simulink model "testing_time_net_3layers"  (R2018b)
settings: Solver=VariableStepAuto  StartTime=0.0  StopTime=10.0  RelTol=1e-3
libraries: neural x97
(part 2 of 6)

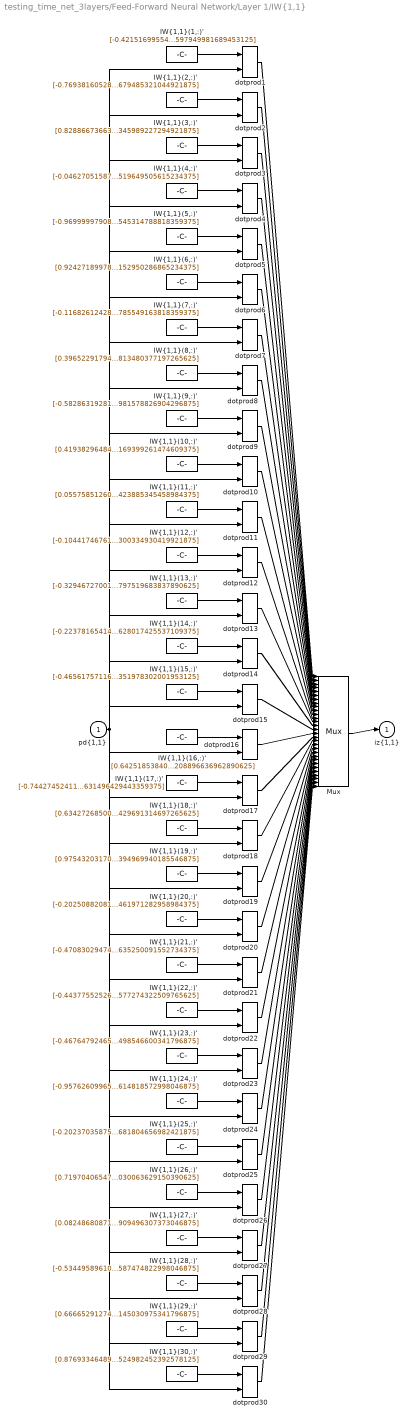
== system testing_time_net_3layers/Feed-Forward Neural Network/Layer 1/IW{1,1} ==
  "pd{1,1}" : Inport  PortDimensions=10
      mask Display: e = 0.06;c1 = [120 230 180]/255;c2 = ([120 230 180]+0)/(256+128);c3 = ([120 230 180]+128)/(256+128);patch([0 1 1 0],[0 0 1 1],c1);patch([0 1 1 1-e 1-e 0+e],[0 0 1 1-e 0+e 0+e],c2);patch([0 0 1 1-e 0+e 0+e],[0 1 1 1-e 1-e 0+e],c3);plot([0 1 1 0 0],[0 0 1 1 0]);
  "IW{1,1}(1,:)'" : Constant  Value=[-0.421516995547151440693056656527915038168430328369140625;-0.78331730650782827041211930918507277965545654296875;0.87573894753330805418300997189362533390522003173828125;0.12417975566875194548543959172093309462070465087890625;-0.1892164229878487702318778929111431352794170379638671875;0.77197968809492589770115955616347491741180419921875;-0.162179356745227154501520772100775502622127532958984375;-0.47501513253533367286962629805202595889568328857421875;0.361899777531295041566039571989676915109157562255859375;-1.0678850199978360269170707397279329597949981689453125]
      mask Display: e = 0.06;c1 = [120 150 230]/255;c2 = ([120 150 230]+0)/383;c3 = ([120 150 230]+128)/383;patch([0 1 1 0],[0 0 1 1],c1);patch([0 1 1 1-e 1-e 0+e],[0 0 1 1-e 0+e 0+e],c2);patch([0 0 1 1-e 0+e 0+e],[0 1 1 1-e 1-e 0+e],c3);plot([0 1 1 0 0],[0 0 1 1 0]);disp('Weights');
  "IW{1,1}(10,:)'" : Constant  Value=[0.419382964847384187567769231463898904621601104736328125;-1.10662440705737896706750689190812408924102783203125;-0.520362222704379373539040898322127759456634521484375;-0.7192359088296094160597249356214888393878936767578125;-1.00725625065982793415741980425082147121429443359375;0.21548425562980089154052620870061218738555908203125;0.381727115430177843524717218315345235168933868408203125;0.04936193217574691427529387510730884969234466552734375;-0.430557268169915463573715896927751600742340087890625;0.22991864804537021083064018966979347169399261474609375]
      mask Display: e = 0.06;c1 = [120 150 230]/255;c2 = ([120 150 230]+0)/383;c3 = ([120 150 230]+128)/383;patch([0 1 1 0],[0 0 1 1],c1);patch([0 1 1 1-e 1-e 0+e],[0 0 1 1-e 0+e 0+e],c2);patch([0 0 1 1-e 0+e 0+e],[0 1 1 1-e 1-e 0+e],c3);plot([0 1 1 0 0],[0 0 1 1 0]);disp('Weights');
  "IW{1,1}(11,:)'" : Constant  Value=[0.055758512605714904974973933349247090518474578857421875;-0.81841828037387120975409970924374647438526153564453125;1.1440676666439248965190245144185610115528106689453125;-0.36136848687608680297245200563338585197925567626953125;-0.86626831394689973731004783985554240643978118896484375;0.0149492584043128019788415627999711432494223117828369140625;-0.048457932577146568819959071561243035830557346343994140625;0.1490262934767860036888720287606702186167240142822265625;-0.2238428092966452676026989365709596313536167144775390625;0.80848234625489057147973426253884099423885345458984375]
      mask Display: e = 0.06;c1 = [120 150 230]/255;c2 = ([120 150 230]+0)/383;c3 = ([120 150 230]+128)/383;patch([0 1 1 0],[0 0 1 1],c1);patch([0 1 1 1-e 1-e 0+e],[0 0 1 1-e 0+e 0+e],c2);patch([0 0 1 1-e 0+e 0+e],[0 1 1 1-e 1-e 0+e],c3);plot([0 1 1 0 0],[0 0 1 1 0]);disp('Weights');
  "IW{1,1}(12,:)'" : Constant  Value=[-0.10441746761245880581459033464852836914360523223876953125;-0.11643946018543309406378938319903681986033916473388671875;0.1902729302910009800964274973011924885213375091552734375;0.469215077641359223914463427718146704137325286865234375;0.06023180084088856911517240178000065498054027557373046875;-1.097601095565966744516117614693939685821533203125;-0.19260021082754497090405720882699824869632720947265625;-0.95631655884358857111493534830515272915363311767578125;0.33607616325035305493429405032657086849212646484375;0.243167221789594101277742765887524001300334930419921875]
      mask Display: e = 0.06;c1 = [120 150 230]/255;c2 = ([120 150 230]+0)/383;c3 = ([120 150 230]+128)/383;patch([0 1 1 0],[0 0 1 1],c1);patch([0 1 1 1-e 1-e 0+e],[0 0 1 1-e 0+e 0+e],c2);patch([0 0 1 1-e 0+e 0+e],[0 1 1 1-e 1-e 0+e],c3);plot([0 1 1 0 0],[0 0 1 1 0]);disp('Weights');
  "IW{1,1}(13,:)'" : Constant  Value=[-0.32946727001318809602281589832273311913013458251953125;-0.59573828714480148160959060987806878983974456787109375;0.047375503865274802561824429858461371622979640960693359375;-0.8972999906601477615453177349991165101528167724609375;0.1344036346182840013785408928015385754406452178955078125;-0.307730158359239336363089023507200181484222412109375;-0.50048527970131839737177870119921863079071044921875;0.5770479702135820065933557998505420982837677001953125;1.0835405192943083907408663435489870607852935791015625;0.00146764010904052756567583770674900733865797519683837890625]
      mask Display: e = 0.06;c1 = [120 150 230]/255;c2 = ([120 150 230]+0)/383;c3 = ([120 150 230]+128)/383;patch([0 1 1 0],[0 0 1 1],c1);patch([0 1 1 1-e 1-e 0+e],[0 0 1 1-e 0+e 0+e],c2);patch([0 0 1 1-e 0+e 0+e],[0 1 1 1-e 1-e 0+e],c3);plot([0 1 1 0 0],[0 0 1 1 0]);disp('Weights');
  "IW{1,1}(14,:)'" : Constant  Value=[-0.2237816541400211300949507631230517290532588958740234375;-0.2255117106004860261236899532377719879150390625;0.66053775807437242750808081837021745741367340087890625;-0.271471723530878839003577240873710252344608306884765625;-0.275504989896624030709659791682497598230838775634765625;1.090081336576464554610765844699926674365997314453125;-1.0836555650409618323237737058661878108978271484375;0.4045819957397511767993592002312652766704559326171875;-0.38831379318925274279905579533078707754611968994140625;0.81705807101285576887761408215737901628017425537109375]
      mask Display: e = 0.06;c1 = [120 150 230]/255;c2 = ([120 150 230]+0)/383;c3 = ([120 150 230]+128)/383;patch([0 1 1 0],[0 0 1 1],c1);patch([0 1 1 1-e 1-e 0+e],[0 0 1 1-e 0+e 0+e],c2);patch([0 0 1 1-e 0+e 0+e],[0 1 1 1-e 1-e 0+e],c3);plot([0 1 1 0 0],[0 0 1 1 0]);disp('Weights');
  "IW{1,1}(15,:)'" : Constant  Value=[-0.465617571164088916990664301920332945883274078369140625;0.20021971547416994585688598817796446382999420166015625;-0.866762424370275397222940227948129177093505859375;-1.15028928445346334541454780264757573604583740234375;0.51764057051554213106925317333661951124668121337890625;0.308597669704476273988547063709120266139507293701171875;-0.37399670770951420895045202996698208153247833251953125;-0.398601119454665531183223947664373554289340972900390625;1.0574802584945477423872262079385109245777130126953125;0.33715076808321076118346582006779499351978302001953125]
      mask Display: e = 0.06;c1 = [120 150 230]/255;c2 = ([120 150 230]+0)/383;c3 = ([120 150 230]+128)/383;patch([0 1 1 0],[0 0 1 1],c1);patch([0 1 1 1-e 1-e 0+e],[0 0 1 1-e 0+e 0+e],c2);patch([0 0 1 1-e 0+e 0+e],[0 1 1 1-e 1-e 0+e],c3);plot([0 1 1 0 0],[0 0 1 1 0]);disp('Weights');
  "IW{1,1}(16,:)'" : Constant  Value=[0.64251853840130268569197369288303889334201812744140625;-0.9103176888822288592706399867893196642398834228515625;0.86486580306804949902499402014655061066150665283203125;-0.802804038444044021360923579777590930461883544921875;-0.0306119017760589258447811999985788133926689624786376953125;0.48642105708010030529209188898676075041294097900390625;-0.32892673265715888231142116637784056365489959716796875;-0.33398839064729857195601425701170228421688079833984375;0.49490021343151535671012197781237773597240447998046875;-0.66415276437832526656990239644073881208896636962890625]
      mask Display: e = 0.06;c1 = [120 150 230]/255;c2 = ([120 150 230]+0)/383;c3 = ([120 150 230]+128)/383;patch([0 1 1 0],[0 0 1 1],c1);patch([0 1 1 1-e 1-e 0+e],[0 0 1 1-e 0+e 0+e],c2);patch([0 0 1 1-e 0+e 0+e],[0 1 1 1-e 1-e 0+e],c3);plot([0 1 1 0 0],[0 0 1 1 0]);disp('Weights');
  "IW{1,1}(17,:)'" : Constant  Value=[-0.7442745241102250997045075564528815448284149169921875;0.8528849176435795431672204358619637787342071533203125;0.1472831429426426919082615540901315398514270782470703125;0.70582238257419860349983764535863883793354034423828125;0.71412598991594522512826870297431014478206634521484375;0.72628375847696113876139634157880209386348724365234375;0.1256024263367492010967652049657772295176982879638671875;-0.46946656479521109428532099627773277461528778076171875;-1.0040813607858349865153968494269065558910369873046875;-0.2292580558718129990491974012911668978631496429443359375]
      mask Display: e = 0.06;c1 = [120 150 230]/255;c2 = ([120 150 230]+0)/383;c3 = ([120 150 230]+128)/383;patch([0 1 1 0],[0 0 1 1],c1);patch([0 1 1 1-e 1-e 0+e],[0 0 1 1-e 0+e 0+e],c2);patch([0 0 1 1-e 0+e 0+e],[0 1 1 1-e 1-e 0+e],c3);plot([0 1 1 0 0],[0 0 1 1 0]);disp('Weights');
  "IW{1,1}(18,:)'" : Constant  Value=[0.63427268500540068263404691606410779058933258056640625;0.59103300526930524494417795722256414592266082763671875;-0.86930498564431835095689393710927106440067291259765625;0.47010501751860600538890366806299425661563873291015625;0.01107508729048142966100432005305265192873775959014892578125;-0.2436611852579689541098417748798965476453304290771484375;0.59770169939745343423709300623158924281597137451171875;-0.56273298477798416872275311106932349503040313720703125;0.52803737767482206155733592822798527777194976806640625;-0.84961313470226207389401906766579486429691314697265625]
      mask Display: e = 0.06;c1 = [120 150 230]/255;c2 = ([120 150 230]+0)/383;c3 = ([120 150 230]+128)/383;patch([0 1 1 0],[0 0 1 1],c1);patch([0 1 1 1-e 1-e 0+e],[0 0 1 1-e 0+e 0+e],c2);patch([0 0 1 1-e 0+e 0+e],[0 1 1 1-e 1-e 0+e],c3);plot([0 1 1 0 0],[0 0 1 1 0]);disp('Weights');
  "IW{1,1}(19,:)'" : Constant  Value=[0.975432031709934310725884643034078180789947509765625;-0.97599556091563943738265152205713093280792236328125;-0.6895423113845835505486547845066525042057037353515625;0.84075064756283790501356634194962680339813232421875;-0.383314027564946258053169003687798976898193359375;0.62542572352496639265240219174302183091640472412109375;0.266943736307111156857985179158276878297328948974609375;-0.392637618319390480081665373290888965129852294921875;0.447913641889938485274313961781444959342479705810546875;0.102248576506790367357524473845842294394969940185546875]
      mask Display: e = 0.06;c1 = [120 150 230]/255;c2 = ([120 150 230]+0)/383;c3 = ([120 150 230]+128)/383;patch([0 1 1 0],[0 0 1 1],c1);patch([0 1 1 1-e 1-e 0+e],[0 0 1 1-e 0+e 0+e],c2);patch([0 0 1 1-e 0+e 0+e],[0 1 1 1-e 1-e 0+e],c3);plot([0 1 1 0 0],[0 0 1 1 0]);disp('Weights');
  "IW{1,1}(2,:)'" : Constant  Value=[-0.76938160528967503015707052327343262732028961181640625;0.7862566691334504920263270832947455346584320068359375;-0.81420490348209995090655866079032421112060546875;-0.204713576431253263532283881431794725358486175537109375;-0.55612978133927970514349681252497248351573944091796875;0.72815871682461885683323998819105327129364013671875;0.04013221143393431999957243760945857502520084381103515625;-0.9673622952210880754364552558399736881256103515625;0.40640017773961523150916264057741500437259674072265625;-0.10349116011036833817637869969985331408679485321044921875]
      mask Display: e = 0.06;c1 = [120 150 230]/255;c2 = ([120 150 230]+0)/383;c3 = ([120 150 230]+128)/383;patch([0 1 1 0],[0 0 1 1],c1);patch([0 1 1 1-e 1-e 0+e],[0 0 1 1-e 0+e 0+e],c2);patch([0 0 1 1-e 0+e 0+e],[0 1 1 1-e 1-e 0+e],c3);plot([0 1 1 0 0],[0 0 1 1 0]);disp('Weights');
  "IW{1,1}(20,:)'" : Constant  Value=[-0.2025088208162877656537403936454211361706256866455078125;-0.57236234131093122190492294976138509809970855712890625;-0.327308764956311393223842287625302560627460479736328125;0.822894315456416780563131396775133907794952392578125;-0.65739164958324114440557650596019811928272247314453125;0.904731349381545424392925269785337150096893310546875;0.435151068218643521934296813924447633326053619384765625;0.33316747742229935180802158356527797877788543701171875;0.10353128021030648386879846611918765120208263397216796875;0.76559551711986217892302875043242238461971282958984375]
      mask Display: e = 0.06;c1 = [120 150 230]/255;c2 = ([120 150 230]+0)/383;c3 = ([120 150 230]+128)/383;patch([0 1 1 0],[0 0 1 1],c1);patch([0 1 1 1-e 1-e 0+e],[0 0 1 1-e 0+e 0+e],c2);patch([0 0 1 1-e 0+e 0+e],[0 1 1 1-e 1-e 0+e],c3);plot([0 1 1 0 0],[0 0 1 1 0]);disp('Weights');
  "IW{1,1}(21,:)'" : Constant  Value=[-0.47083029474935778058153346137260086834430694580078125;-0.7041358974756082300672233031946234405040740966796875;-0.80111168228982176930941250247997231781482696533203125;0.331821973680829829245197970521985553205013275146484375;0.83064205981245320398187459431937895715236663818359375;-0.1664533857760358281918655620756908319890499114990234375;-0.0145485423815401061775620661364882835187017917633056640625;-0.54452016713101947242847700181300751864910125732421875;-0.28983744411975764787570142289041541516780853271484375;-0.94844892993595431018860608674003742635250091552734375]
      mask Display: e = 0.06;c1 = [120 150 230]/255;c2 = ([120 150 230]+0)/383;c3 = ([120 150 230]+128)/383;patch([0 1 1 0],[0 0 1 1],c1);patch([0 1 1 1-e 1-e 0+e],[0 0 1 1-e 0+e 0+e],c2);patch([0 0 1 1-e 0+e 0+e],[0 1 1 1-e 1-e 0+e],c3);plot([0 1 1 0 0],[0 0 1 1 0]);disp('Weights');
  "IW{1,1}(22,:)'" : Constant  Value=[-0.44377552526932595444719709121272899210453033447265625;0.19874440469811560650015280771185643970966339111328125;0.5171798378338021695554971302044577896595001220703125;-0.5948167380925024616544760647229850292205810546875;-0.51803140394908064880752363023930229246616363525390625;0.1768730574972974534109226851796847768127918243408203125;0.80343393299311960387143471962190233170986175537109375;-0.8062398440105464914040567236952483654022216796875;-0.465132085706827347326708377295290119946002960205078125;1.03650226090022190561512616113759577274322509765625]
      mask Display: e = 0.06;c1 = [120 150 230]/255;c2 = ([120 150 230]+0)/383;c3 = ([120 150 230]+128)/383;patch([0 1 1 0],[0 0 1 1],c1);patch([0 1 1 1-e 1-e 0+e],[0 0 1 1-e 0+e 0+e],c2);patch([0 0 1 1-e 0+e 0+e],[0 1 1 1-e 1-e 0+e],c3);plot([0 1 1 0 0],[0 0 1 1 0]);disp('Weights');
  "IW{1,1}(23,:)'" : Constant  Value=[-0.46764792465058169224079165360308252274990081787109375;0.50005215197359598189308371729566715657711029052734375;-0.88978890911745145420042035766527988016605377197265625;-0.80418845225870783099964000939507968723773956298828125;0.6806653554057879862426716499612666666507720947265625;0.295185022260585572251301300639170221984386444091796875;-0.07390143313321236029356242624999140389263629913330078125;-0.056131327503942486656374200038044364191591739654541015625;-0.8360482319812678753123691421933472156524658203125;-0.6039061531303377972079715618747286498546600341796875]
      mask Display: e = 0.06;c1 = [120 150 230]/255;c2 = ([120 150 230]+0)/383;c3 = ([120 150 230]+128)/383;patch([0 1 1 0],[0 0 1 1],c1);patch([0 1 1 1-e 1-e 0+e],[0 0 1 1-e 0+e 0+e],c2);patch([0 0 1 1-e 0+e 0+e],[0 1 1 1-e 1-e 0+e],c3);plot([0 1 1 0 0],[0 0 1 1 0]);disp('Weights');
  "IW{1,1}(24,:)'" : Constant  Value=[-0.95762609965604872375166678466484881937503814697265625;0.65438594435912833535695654063601978123188018798828125;-0.1242314911165121049663184749078936874866485595703125;0.741863364861050200715908431448042392730712890625;-0.0248763192293788883147076518298490555025637149810791015625;-0.049901107492933645393140551504984614439308643341064453125;-0.68711823879287925453951402232632972300052642822265625;-1.0689661379880330827063517062924802303314208984375;-0.1601685256211442254237198312694090418517589569091796875;-0.388585757475137849592528027642401866614818572998046875]
      mask Display: e = 0.06;c1 = [120 150 230]/255;c2 = ([120 150 230]+0)/383;c3 = ([120 150 230]+128)/383;patch([0 1 1 0],[0 0 1 1],c1);patch([0 1 1 1-e 1-e 0+e],[0 0 1 1-e 0+e 0+e],c2);patch([0 0 1 1-e 0+e 0+e],[0 1 1 1-e 1-e 0+e],c3);plot([0 1 1 0 0],[0 0 1 1 0]);disp('Weights');
  "IW{1,1}(25,:)'" : Constant  Value=[-0.2023703587521977487195812273057526908814907073974609375;-0.78834111774768145242120453985990025103092193603515625;-0.056082359669903943111268773691335809417068958282470703125;0.7680098070380834140991055392078123986721038818359375;-0.47361396685274448348224041183129884302616119384765625;-0.97947942318078295986794046257273294031620025634765625;0.42643292657888576258073953795246779918670654296875;-0.25973662139739672749527699124882929027080535888671875;0.352780333259110123744761722264229319989681243896484375;-0.76057665100687898984688217751681804656982421875]
      mask Display: e = 0.06;c1 = [120 150 230]/255;c2 = ([120 150 230]+0)/383;c3 = ([120 150 230]+128)/383;patch([0 1 1 0],[0 0 1 1],c1);patch([0 1 1 1-e 1-e 0+e],[0 0 1 1-e 0+e 0+e],c2);patch([0 0 1 1-e 0+e 0+e],[0 1 1 1-e 1-e 0+e],c3);plot([0 1 1 0 0],[0 0 1 1 0]);disp('Weights');
  "IW{1,1}(26,:)'" : Constant  Value=[0.71970406547438015021356250144890509545803070068359375;0.93388981552474670255747923874878324568271636962890625;-0.54894473444162772413079665057011879980564117431640625;0.1602146385281348062168405022021033801138401031494140625;0.2145369956237772601781443881918676197528839111328125;-0.585766950119024354393104658811353147029876708984375;0.1146544013505880477143961115871206857264041900634765625;-0.9116817411373097090887540616677142679691314697265625;0.1305499485880995680364691224895068444311618804931640625;-0.8266585341918588625276242964901030063629150390625]
      mask Display: e = 0.06;c1 = [120 150 230]/255;c2 = ([120 150 230]+0)/383;c3 = ([120 150 230]+128)/383;patch([0 1 1 0],[0 0 1 1],c1);patch([0 1 1 1-e 1-e 0+e],[0 0 1 1-e 0+e 0+e],c2);patch([0 0 1 1-e 0+e 0+e],[0 1 1 1-e 1-e 0+e],c3);plot([0 1 1 0 0],[0 0 1 1 0]);disp('Weights');
  "IW{1,1}(27,:)'" : Constant  Value=[0.0824868087151008622104342293823719955980777740478515625;-0.08051288002138813626462621186874457634985446929931640625;0.19252569566822630431346397017478011548519134521484375;0.62584288924756226180079465848393738269805908203125;-1.5154080094857531602059452779940329492092132568359375;-0.32059707297645712031908260541968047618865966796875;0.14521227413854698173878432498895563185214996337890625;0.62618251370211386319653001919505186378955841064453125;-0.30611424035098566687196353086619637906551361083984375;-0.10460790403111978885686284002076718024909496307373046875]
      mask Display: e = 0.06;c1 = [120 150 230]/255;c2 = ([120 150 230]+0)/383;c3 = ([120 150 230]+128)/383;patch([0 1 1 0],[0 0 1 1],c1);patch([0 1 1 1-e 1-e 0+e],[0 0 1 1-e 0+e 0+e],c2);patch([0 0 1 1-e 0+e 0+e],[0 1 1 1-e 1-e 0+e],c3);plot([0 1 1 0 0],[0 0 1 1 0]);disp('Weights');
  "IW{1,1}(28,:)'" : Constant  Value=[-0.53449589610124126348722484181053005158901214599609375;-0.81070213464066653852313493189285509288311004638671875;-0.39600805216664503038970224224613048136234283447265625;-0.56368934652596236478672153680236078798770904541015625;-0.71656916746642773663467096412205137312412261962890625;-0.8126551125729495339555796817876398563385009765625;-0.1102646818088157953940964262073975987732410430908203125;-0.1412722588335082185562185941307689063251018524169921875;0.801303604206889730221519130282104015350341796875;-0.270353860735323248132289108980330638587474822998046875]
      mask Display: e = 0.06;c1 = [120 150 230]/255;c2 = ([120 150 230]+0)/383;c3 = ([120 150 230]+128)/383;patch([0 1 1 0],[0 0 1 1],c1);patch([0 1 1 1-e 1-e 0+e],[0 0 1 1-e 0+e 0+e],c2);patch([0 0 1 1-e 0+e 0+e],[0 1 1 1-e 1-e 0+e],c3);plot([0 1 1 0 0],[0 0 1 1 0]);disp('Weights');
  "IW{1,1}(29,:)'" : Constant  Value=[0.66665291274113991359939745962037704885005950927734375;-0.57326133429640113714498284025467000901699066162109375;0.8646031256409176801724925098824314773082733154296875;0.63432518432133921937321474615600891411304473876953125;0.83723629990477121953773576024104841053485870361328125;0.491305384109994747188210340027580969035625457763671875;-0.187127791256418263277083724460680969059467315673828125;0.15303927921905791098566851360374130308628082275390625;-0.2370470527101120328250516422485816292464733123779296875;-0.839340070514452918359893374145030975341796875]
      mask Display: e = 0.06;c1 = [120 150 230]/255;c2 = ([120 150 230]+0)/383;c3 = ([120 150 230]+128)/383;patch([0 1 1 0],[0 0 1 1],c1);patch([0 1 1 1-e 1-e 0+e],[0 0 1 1-e 0+e 0+e],c2);patch([0 0 1 1-e 0+e 0+e],[0 1 1 1-e 1-e 0+e],c3);plot([0 1 1 0 0],[0 0 1 1 0]);disp('Weights');
  "IW{1,1}(3,:)'" : Constant  Value=[0.8288667366318114293477492537931539118289947509765625;-0.76876764428917809812702444105525501072406768798828125;-0.373574167176615679064610731074935756623744964599609375;-0.32630623855510820785497116958140395581722259521484375;0.05280441495481154323687889018401619978249073028564453125;0.480377421896862000227912403715890832245349884033203125;0.267266292755837520100925530641688965260982513427734375;1.05969396714446162377498694695532321929931640625;-0.56255390999751087033331486964016221463680267333984375;0.52295111090456725122521675075404345989227294921875]
      mask Display: e = 0.06;c1 = [120 150 230]/255;c2 = ([120 150 230]+0)/383;c3 = ([120 150 230]+128)/383;patch([0 1 1 0],[0 0 1 1],c1);patch([0 1 1 1-e 1-e 0+e],[0 0 1 1-e 0+e 0+e],c2);patch([0 0 1 1-e 0+e 0+e],[0 1 1 1-e 1-e 0+e],c3);plot([0 1 1 0 0],[0 0 1 1 0]);disp('Weights');
  "IW{1,1}(30,:)'" : Constant  Value=[0.87693346489520662689898244934738613665103912353515625;-0.43086221404642766064085890320711769163608551025390625;-0.82120426980066429933913241256959736347198486328125;0.7489828074122704126835969873354770243167877197265625;0.57819877940140518290945692569948732852935791015625;-0.70593444630110535609190947070601396262645721435546875;-0.63536853888569522208484841030440293252468109130859375;0.2225665376333621214843816460415837354958057403564453125;0.621290406365510694541853808914311230182647705078125;0.0018887641765197968508893655581459825043566524982452392578125]
      mask Display: e = 0.06;c1 = [120 150 230]/255;c2 = ([120 150 230]+0)/383;c3 = ([120 150 230]+128)/383;patch([0 1 1 0],[0 0 1 1],c1);patch([0 1 1 1-e 1-e 0+e],[0 0 1 1-e 0+e 0+e],c2);patch([0 0 1 1-e 0+e 0+e],[0 1 1 1-e 1-e 0+e],c3);plot([0 1 1 0 0],[0 0 1 1 0]);disp('Weights');
  "IW{1,1}(4,:)'" : Constant  Value=[-0.0462705158743447475533372426070854999125003814697265625;-0.072884328013425536685332417619065381586551666259765625;0.489054660084421277677080297507927753031253814697265625;-1.0852254774048615271198059417656622827053070068359375;0.445748203646976370873034056785400025546550750732421875;0.64111660070044462766958304200670681893825531005859375;-0.200855870194340202505856041170773096382617950439453125;0.2263966967951359376964859393410733900964260101318359375;-0.9795630210186663244797955485410057008266448974609375;0.50338011586868824931428889613016508519649505615234375]
      mask Display: e = 0.06;c1 = [120 150 230]/255;c2 = ([120 150 230]+0)/383;c3 = ([120 150 230]+128)/383;patch([0 1 1 0],[0 0 1 1],c1);patch([0 1 1 1-e 1-e 0+e],[0 0 1 1-e 0+e 0+e],c2);patch([0 0 1 1-e 0+e 0+e],[0 1 1 1-e 1-e 0+e],c3);plot([0 1 1 0 0],[0 0 1 1 0]);disp('Weights');
  "IW{1,1}(5,:)'" : Constant  Value=[-0.96999997908646806710208920776494778692722320556640625;-0.267611644730110176393367282798863016068935394287109375;0.6178107533447489974065547357895411550998687744140625;0.333743992432052161145605850833817385137081146240234375;0.70935017114413068117784177957219071686267852783203125;0.336152790660474043438199487354722805321216583251953125;-0.91294133818778100408763975792680867016315460205078125;0.7804425482838919236883157282136380672454833984375;0.346469939746774924227423753109178505837917327880859375;-0.0499996701565888768126200147889903746545314788818359375]
      mask Display: e = 0.06;c1 = [120 150 230]/255;c2 = ([120 150 230]+0)/383;c3 = ([120 150 230]+128)/383;patch([0 1 1 0],[0 0 1 1],c1);patch([0 1 1 1-e 1-e 0+e],[0 0 1 1-e 0+e 0+e],c2);patch([0 0 1 1-e 0+e 0+e],[0 1 1 1-e 1-e 0+e],c3);plot([0 1 1 0 0],[0 0 1 1 0]);disp('Weights');
  "IW{1,1}(6,:)'" : Constant  Value=[0.92427189978005619419576532891369424760341644287109375;-0.150812147743339786121197221291367895901203155517578125;-1.0929626212993921452465428956202231347560882568359375;-0.00836315481885591648081312854401403455995023250579833984375;0.95836162423276061161914185504429042339324951171875;-0.74490512357986504721196752143441699445247650146484375;-0.528324445751827465045380449737422168254852294921875;-0.2266839625006198122303402442412334494292736053466796875;-0.35328934440316428489126110434881411492824554443359375;0.2114311775140543525619563069994910620152950286865234375]
      mask Display: e = 0.06;c1 = [120 150 230]/255;c2 = ([120 150 230]+0)/383;c3 = ([120 150 230]+128)/383;patch([0 1 1 0],[0 0 1 1],c1);patch([0 1 1 1-e 1-e 0+e],[0 0 1 1-e 0+e 0+e],c2);patch([0 0 1 1-e 0+e 0+e],[0 1 1 1-e 1-e 0+e],c3);plot([0 1 1 0 0],[0 0 1 1 0]);disp('Weights');
  "IW{1,1}(7,:)'" : Constant  Value=[-0.11682612428154361128296301330919959582388401031494140625;-0.398365834958046394209674190278747119009494781494140625;0.65463313513670318144477278110571205615997314453125;0.516167801840001327917661910760216414928436279296875;-0.72892699168909624862777718590223230421543121337890625;0.06821628645151341097108144140293006785213947296142578125;-0.91732870467362215283202431237441487610340118408203125;-0.2341193843690918818811752544206683523952960968017578125;0.91563825655990849217147342642419971525669097900390625;0.61258959061783568866843552314094267785549163818359375]
      mask Display: e = 0.06;c1 = [120 150 230]/255;c2 = ([120 150 230]+0)/383;c3 = ([120 150 230]+128)/383;patch([0 1 1 0],[0 0 1 1],c1);patch([0 1 1 1-e 1-e 0+e],[0 0 1 1-e 0+e 0+e],c2);patch([0 0 1 1-e 0+e 0+e],[0 1 1 1-e 1-e 0+e],c3);plot([0 1 1 0 0],[0 0 1 1 0]);disp('Weights');
  "IW{1,1}(8,:)'" : Constant  Value=[0.39652291794354532772359789305482991039752960205078125;-0.8191322822151259064327177839004434645175933837890625;-0.9377644294755673737284951130277477204799652099609375;0.69420630420340445621008029775111936032772064208984375;0.366796876324141207792450813940376974642276763916015625;0.601584285943538521479467817698605358600616455078125;0.4726380306486921423214653259492479264736175537109375;0.053742608808895551975037818692726432345807552337646484375;-0.380569436779539527204718751818290911614894866943359375;0.6358365241199896988888440318987704813480377197265625]
      mask Display: e = 0.06;c1 = [120 150 230]/255;c2 = ([120 150 230]+0)/383;c3 = ([120 150 230]+128)/383;patch([0 1 1 0],[0 0 1 1],c1);patch([0 1 1 1-e 1-e 0+e],[0 0 1 1-e 0+e 0+e],c2);patch([0 0 1 1-e 0+e 0+e],[0 1 1 1-e 1-e 0+e],c3);plot([0 1 1 0 0],[0 0 1 1 0]);disp('Weights');
  "IW{1,1}(9,:)'" : Constant  Value=[-0.58286319281235476896796399159939028322696685791015625;0.376414497405152703723985041506239213049411773681640625;-0.404600224190247492739302970221615396440029144287109375;-0.47847635461064286221954944267054088413715362548828125;-0.651979234115994898957069381140172481536865234375;-1.1841161345613500088802538812160491943359375;-0.20080269007832318717277075847960077226161956787109375;0.2197030461064573836349467228501453064382076263427734375;0.52467276699675491347107936235261149704456329345703125;-0.409134638386210613969495852870750240981578826904296875]
      mask Display: e = 0.06;c1 = [120 150 230]/255;c2 = ([120 150 230]+0)/383;c3 = ([120 150 230]+128)/383;patch([0 1 1 0],[0 0 1 1],c1);patch([0 1 1 1-e 1-e 0+e],[0 0 1 1-e 0+e 0+e],c2);patch([0 0 1 1-e 0+e 0+e],[0 1 1 1-e 1-e 0+e],c3);plot([0 1 1 0 0],[0 0 1 1 0]);disp('Weights');
  Mux : Mux  Inputs=30
      mask Display: e = 0.06;c1 = [120 150 230]/255;c2 = ([120 150 230]+0)/383;c3 = ([120 150 230]+128)/383;patch([0 1 1 0],[0 0 1 1],c1);patch([0 1 1 1-e 1-e 0+e],[0 0 1 1-e 0+e 0+e],c2);patch([0 0 1 1-e 0+e 0+e],[0 1 1 1-e 1-e 0+e],c3);plot([0 1 1 0 0],[0 0 1 1 0]);disp('Mux');
  dotprod{1..30} (30 alike) : neural/Weight Functions/dotprod
  "iz{1,1}" : Outport
      mask Display: e = 0.06;c1 = [120 230 180]/255;c2 = ([120 230 180]+0)/(256+128);c3 = ([120 230 180]+128)/(256+128);patch([0 1 1 0],[0 0 1 1],c1);patch([0 1 1 1-e 1-e 0+e],[0 0 1 1-e 0+e 0+e],c2);patch([0 0 1 1-e 0+e 0+e],[0 1 1 1-e 1-e 0+e],c3);plot([0 1 1 0 0],[0 0 1 1 0]);
  wires:
  "IW{1,1}(1,:)'"/1 -> dotprod1/1
  "pd{1,1}"/1 -> dotprod1/2, dotprod2/2, dotprod3/2, dotprod4/2, dotprod5/2, dotprod6/2, dotprod7/2, dotprod8/2, dotprod9/2, dotprod10/2, dotprod11/2, dotprod12/2, dotprod13/2, dotprod14/2, dotprod15/2, dotprod16/2, dotprod17/2, dotprod18/2, dotprod19/2, dotprod20/2, dotprod21/2, dotprod22/2, dotprod23/2, dotprod24/2, dotprod25/2, dotprod26/2, dotprod27/2, dotprod28/2, dotprod29/2, dotprod30/2
  dotprod1/1 -> Mux/1
  "IW{1,1}(2,:)'"/1 -> dotprod2/1
  dotprod2/1 -> Mux/2
  "IW{1,1}(3,:)'"/1 -> dotprod3/1
  dotprod3/1 -> Mux/3
  "IW{1,1}(4,:)'"/1 -> dotprod4/1
  dotprod4/1 -> Mux/4
  "IW{1,1}(5,:)'"/1 -> dotprod5/1
  dotprod5/1 -> Mux/5
  "IW{1,1}(6,:)'"/1 -> dotprod6/1
  dotprod6/1 -> Mux/6
  "IW{1,1}(7,:)'"/1 -> dotprod7/1
  dotprod7/1 -> Mux/7
  "IW{1,1}(8,:)'"/1 -> dotprod8/1
  dotprod8/1 -> Mux/8
  "IW{1,1}(9,:)'"/1 -> dotprod9/1
  dotprod9/1 -> Mux/9
  "IW{1,1}(10,:)'"/1 -> dotprod10/1
  dotprod10/1 -> Mux/10
  "IW{1,1}(11,:)'"/1 -> dotprod11/1
  dotprod11/1 -> Mux/11
  "IW{1,1}(12,:)'"/1 -> dotprod12/1
  dotprod12/1 -> Mux/12
  "IW{1,1}(13,:)'"/1 -> dotprod13/1
  dotprod13/1 -> Mux/13
  "IW{1,1}(14,:)'"/1 -> dotprod14/1
  dotprod14/1 -> Mux/14
  "IW{1,1}(15,:)'"/1 -> dotprod15/1
  dotprod15/1 -> Mux/15
  "IW{1,1}(16,:)'"/1 -> dotprod16/1
  dotprod16/1 -> Mux/16
  "IW{1,1}(17,:)'"/1 -> dotprod17/1
  dotprod17/1 -> Mux/17
  "IW{1,1}(18,:)'"/1 -> dotprod18/1
  dotprod18/1 -> Mux/18
  "IW{1,1}(19,:)'"/1 -> dotprod19/1
  dotprod19/1 -> Mux/19
  "IW{1,1}(20,:)'"/1 -> dotprod20/1
  dotprod20/1 -> Mux/20
  "IW{1,1}(21,:)'"/1 -> dotprod21/1
  dotprod21/1 -> Mux/21
  "IW{1,1}(22,:)'"/1 -> dotprod22/1
  dotprod22/1 -> Mux/22
  "IW{1,1}(23,:)'"/1 -> dotprod23/1
  dotprod23/1 -> Mux/23
  "IW{1,1}(24,:)'"/1 -> dotprod24/1
  dotprod24/1 -> Mux/24
  "IW{1,1}(25,:)'"/1 -> dotprod25/1
  dotprod25/1 -> Mux/25
  "IW{1,1}(26,:)'"/1 -> dotprod26/1
  dotprod26/1 -> Mux/26
  "IW{1,1}(27,:)'"/1 -> dotprod27/1
  dotprod27/1 -> Mux/27
  "IW{1,1}(28,:)'"/1 -> dotprod28/1
  dotprod28/1 -> Mux/28
  "IW{1,1}(29,:)'"/1 -> dotprod29/1
  dotprod29/1 -> Mux/29
  "IW{1,1}(30,:)'"/1 -> dotprod30/1
  dotprod30/1 -> Mux/30
  Mux/1 -> "iz{1,1}"/1

== system testing_time_net_3layers/Feed-Forward Neural Network/Layer 2/Delays 1 ==
  "p{2}" : Inport  PortDimensions=30
      mask Display: e = 0.06;c1 = [120 230 180]/255;c2 = ([120 230 180]+0)/(256+128);c3 = ([120 230 180]+128)/(256+128);patch([0 1 1 0],[0 0 1 1],c1);patch([0 1 1 1-e 1-e 0+e],[0 0 1 1-e 0+e 0+e],c2);patch([0 0 1 1-e 0+e 0+e],[0 1 1 1-e 1-e 0+e],c3);plot([0 1 1 0 0],[0 0 1 1 0]);
  mux : Mux  Inputs=1
      mask Display: e = 0.06;c1 = [120 150 230]/255;c2 = ([120 150 230]+0)/383;c3 = ([120 150 230]+128)/383;patch([0 1 1 0],[0 0 1 1],c1);patch([0 1 1 1-e 1-e 0+e],[0 0 1 1-e 0+e 0+e],c2);patch([0 0 1 1-e 0+e 0+e],[0 1 1 1-e 1-e 0+e],c3);plot([0 1 1 0 0],[0 0 1 1 0]);disp('Mux')
  "pd{2,1}" : Outport
      mask Display: e = 0.06;c1 = [120 230 180]/255;c2 = ([120 230 180]+0)/(256+128);c3 = ([120 230 180]+128)/(256+128);patch([0 1 1 0],[0 0 1 1],c1);patch([0 1 1 1-e 1-e 0+e],[0 0 1 1-e 0+e 0+e],c2);patch([0 0 1 1-e 0+e 0+e],[0 1 1 1-e 1-e 0+e],c3);plot([0 1 1 0 0],[0 0 1 1 0]);
  wires:
  "p{2}"/1 -> mux/1
  mux/1 -> "pd{2,1}"/1
